simulink model "Ejercicio5_23_03_17"  (R2013a)
settings: Solver=ode45  StartTime=0.0  StopTime=10.0  RelTol=1e-3
libraries: powerlib x23, powerlib_meascontrol x4
settings Model: Creator=Miguel  LastModifiedBy=Miguel

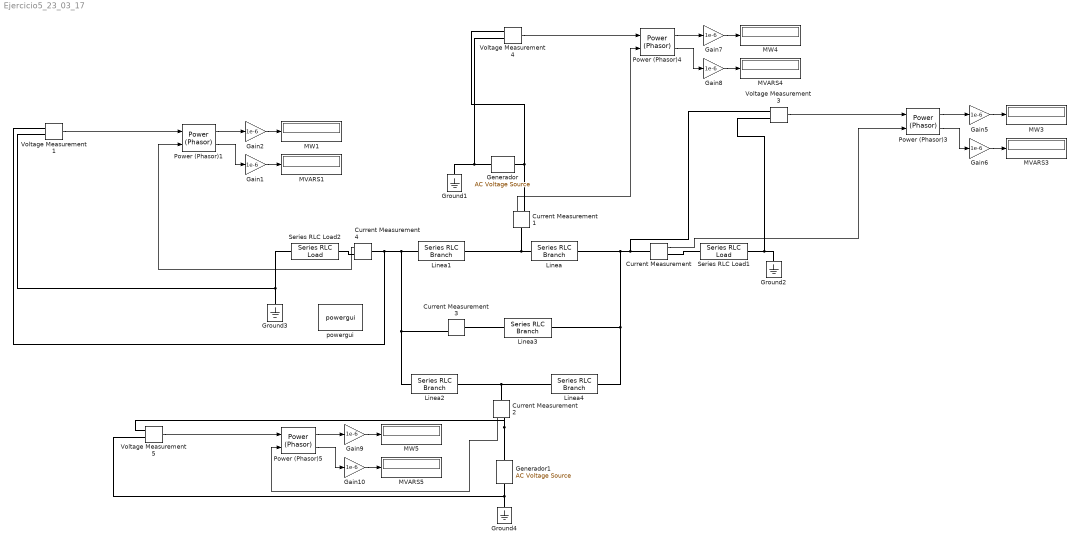
== system Ejercicio5_23_03_17 ==
  Current Measurement{,1..4} (5 alike) : powerlib/Measurements/Current Measurement  PhasorSimulation=on  OutputType=Complex  PSBequivalent=0
  Gain{1..2,5..10} (8 alike) : Gain  Gain=1e-6
  Generador : powerlib/Electrical Sources/AC Voltage Source  Amplitude=200e3*sqrt(2)  Phase=0  Frequency=60  SampleTime=0  Measurements=None
  Generador1 : powerlib/Electrical Sources/AC Voltage Source  Amplitude=200e3*sqrt(2)  Phase=2.1205  Frequency=60  SampleTime=0  Measurements=None
  Ground{1..4} (4 alike) : powerlib/Elements/Ground  LConnTagsString=a
  Linea : powerlib/Elements/Series RLC Branch  LConnTagsString=__new0  RConnTagsString=__new0  BranchType=RL  Resistance=0.1*400  Inductance=0.4*400/(2*pi*60)  SetiL0=off  InitialCurrent=0  Capacitance=1e-6  Setx0=off  InitialVoltage=0  Measurements=None
  Linea1 : powerlib/Elements/Series RLC Branch  LConnTagsString=__new0  RConnTagsString=__new0  BranchType=RL  Resistance=0.5*400  Inductance=0.2*400/(2*pi*60)  SetiL0=off  InitialCurrent=0  Capacitance=1e-6  Setx0=off  InitialVoltage=0  Measurements=None
  Linea2 : powerlib/Elements/Series RLC Branch  LConnTagsString=__new0  RConnTagsString=__new0  BranchType=RL  Resistance=0.5*400  Inductance=0.2*400/(2*pi*60)  SetiL0=off  InitialCurrent=0  Capacitance=1e-6  Setx0=off  InitialVoltage=0  Measurements=None
  Linea3 : powerlib/Elements/Series RLC Branch  LConnTagsString=__new0  RConnTagsString=__new0  BranchType=RL  Resistance=0.1*400  Inductance=0.4*400/(2*pi*60)  SetiL0=off  InitialCurrent=0  Capacitance=1e-6  Setx0=off  InitialVoltage=0  Measurements=None
  Linea4 : powerlib/Elements/Series RLC Branch  LConnTagsString=__new0  RConnTagsString=__new0  BranchType=RL  Resistance=0.1*400  Inductance=0.5*400/(2*pi*60)  SetiL0=off  InitialCurrent=0  Capacitance=1e-6  Setx0=off  InitialVoltage=0  Measurements=None
  MVARS{1,3..5} (4 alike) : Display
  MW{1,3..5} (4 alike) : Display
  Power (Phasor){1,3..5} (4 alike) : powerlib_meascontrol/Measurements/Power (Phasor)
  Series RLC Load1 : powerlib/Elements/Series RLC Load  LConnTagsString=a  RConnTagsString=__new0  NominalVoltage=0.9269*200e3  NominalFrequency=60  ActivePower=0.3*100e6  InductivePower=0.2*100e6  CapacitivePower=0  Setx0=off  InitialVoltage=0  SetiL0=off  InitialCurrent=0  Measurements=None
  Series RLC Load2 : powerlib/Elements/Series RLC Load  LConnTagsString=a  RConnTagsString=__new0  NominalVoltage=0.9135*200e3  NominalFrequency=60  ActivePower=0.2*100e6  InductivePower=0.15*100e6  CapacitivePower=0  Setx0=off  InitialVoltage=0  SetiL0=off  InitialCurrent=0  Measurements=None
  Voltage Measurement{1,3..5} (4 alike) : powerlib/Measurements/Voltage Measurement  PhasorSimulation=on  OutputType=Complex  PSBequivalent=0
  powergui : powerlib/powergui  Priority=1  SimulationMode=Phasor  SolverType=Tustin  SampleTime=50e-6  frequency=60  SPID=off  DisableSnubberDevices=off  DisableRonSwitches=off  DisableVfSwitches=off  SwTol=0  Interpol=off  DisplayEquations=off  frequencyindice=60  Pbase=100e6  ErrMax=1e-4  Iterations=50  UnitsV=kV  UnitsW=MW  FunctionMessages=off  echomessages=off  HookPort=off  EnableUseOfTLC=off  x0status=blocks  RestoreLinks=warning  ResistiveCurrentMeasurement=off  Frange=[0:2:500]  Ylog=off  Xlog=on  ShowGrid=off  save=off  variable=ZData  ZoomFFT=off  StartTime=0.0  cycles=1  DisplayStyle=1  fundamental=60  FreqAxis=off  MaxFrequency=1000  frequencyindicesteady=1  RmsSteady=2  display=off  Ts=0  methode=off
  wires:
  Power (Phasor)3/1 -> Gain5/1
  Power (Phasor)3/2 -> Gain6/1
  Gain5/1 -> MW3/1
  Gain6/1 -> MVARS3/1
  Voltage Measurement3/1 -> Power (Phasor)3/1
  Power (Phasor)4/1 -> Gain7/1
  Power (Phasor)4/2 -> Gain8/1
  Gain7/1 -> MW4/1
  Gain8/1 -> MVARS4/1
  Voltage Measurement4/1 -> Power (Phasor)4/1
  Power (Phasor)5/1 -> Gain9/1
  Power (Phasor)5/2 -> Gain10/1
  Gain9/1 -> MW5/1
  Gain10/1 -> MVARS5/1
  Voltage Measurement5/1 -> Power (Phasor)5/1
  Current Measurement1/1 -> Power (Phasor)4/2
  Current Measurement/1 -> Power (Phasor)3/2
  Current Measurement2/1 -> Power (Phasor)5/2
  Power (Phasor)1/1 -> Gain2/1
  Power (Phasor)1/2 -> Gain1/1
  Gain2/1 -> MW1/1
  Gain1/1 -> MVARS1/1
  Voltage Measurement1/1 -> Power (Phasor)1/1
  Current Measurement4/1 -> Power (Phasor)1/2
  connections:
  Linea/LConn1 -- Current Measurement1/LConn1 -- Linea1/RConn1
  Current Measurement/LConn1 -- Voltage Measurement3/LConn1 -- Linea4/RConn1 -- Linea3/RConn1 -- Linea/RConn1
  Ground2/LConn1 -- Voltage Measurement3/LConn2 -- Series RLC Load1/RConn1
  Generador/LConn1 -- Voltage Measurement4/LConn2 -- Ground1/LConn1
  Current Measurement/RConn1 -- Series RLC Load1/LConn1
  Linea2/LConn1 -- Current Measurement3/RConn1 -- Voltage Measurement1/LConn1 -- Current Measurement4/LConn1 -- Linea1/LConn1
  Linea4/LConn1 -- Current Measurement2/LConn1 -- Linea2/RConn1
  Generador1/LConn1 -- Ground4/LConn1 -- Voltage Measurement5/LConn2
  Current Measurement1/RConn1 -- Voltage Measurement4/LConn1 -- Generador/RConn1
  Current Measurement2/RConn1 -- Generador1/RConn1 -- Voltage Measurement5/LConn1
  Current Measurement3/LConn1 -- Linea3/LConn1
  Series RLC Load2/LConn1 -- Current Measurement4/RConn1
  Series RLC Load2/RConn1 -- Voltage Measurement1/LConn2 -- Ground3/LConn1
